simulink model "Chatr1"  (R2018b)
settings: Solver=FixedStepDiscrete  StartTime=0.0  StopTime=10.0  RelTol=1e-3
settings Model: Creator=mostafa  LastModifiedBy=mostafa
settings DataIOCC: ReturnWorkspaceOutputs=on
settings OptimizationCC: DefaultParameterBehavior=Inlined  EnhancedBackFolding=on  PassReuseOutputArgsAs=Individual arguments  ZeroExternalMemoryAtStartup=off  ZeroInternalMemoryAtStartup=off  OptimizeBlockOrder=speed  DifferentSizesBufferReuse=on  OptimizationCustomize=off
settings DebuggingCC: UnderspecifiedInitializationDetection=Classic  MergeDetectMultiDrivingBlocksExec=none  ParameterTunabilityLossMsg=error  SFMachineParentedDataDiag=error
settings ModelReferenceCC: PropagateSignalLabelsOutOfModel=off
settings SFSimCC: MATLABDynamicMemAlloc=off
settings RTWCC: SystemTargetFile=ert.tlc  GenCodeOnly=on  TemplateMakefile=ert_default_tmf  GenerateReport=on  IncludeHyperlinkInReport=on  LaunchReport=on  GenerateTraceInfo=on  GenerateTraceReport=on  GenerateTraceReportSl=on  GenerateTraceReportSf=on  GenerateTraceReportEml=on
settings CodeAppCC: ForceParamTrailComments=on  IgnoreCustomStorageClasses=off  OperatorAnnotations=on  SimulinkDataObjDesc=on  SFDataObjDesc=on  InsertBlockDesc=on  StateflowObjectComments=on
settings ERTTargetCC: TargetLangStandard=C99 (ISO)  GenerateSampleERTMain=on  InlinedParameterPlacement=NonHierarchical  ERTCustomFileTemplate=example_file_process.tlc

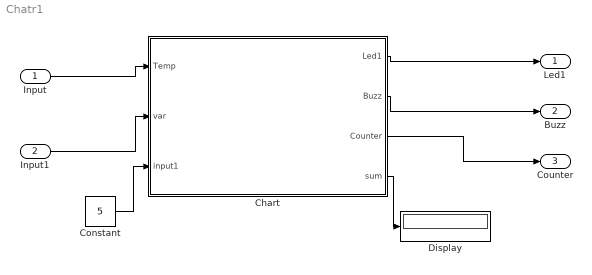
== system Chatr1 ==
  Input : Inport
  Input1 : Inport  Port=2
  Chart : Stateflow chart  TreatAsAtomicUnit=on
  Constant : Constant  Value=5  VectorParams1D=off  OutDataTypeStr=uint8
  Display : Display
  "Led1 " : Outport
  Buzz : Outport  Port=2
  Counter : Outport  Port=3
  wires:
  Chart/1(Led1) -> "Led1 "/1
  Chart/2(Buzz) -> Buzz/1
  Input/1 -> Chart/1(Temp)
  Input1/1 -> Chart/2(var)
  Chart/3(Counter) -> Counter/1
  Constant/1 -> Chart/3(input1)
  Chart/4(sum) -> Display/1

== stateflow chart Chatr1/Chart ==
  note: Do not put any code along
      | the transitions that run
      | down the right side!
  state AlarmOff [commented out]
    en:
    % initialize
    Offcounter=0;
    du:
    Led1 =0;
    Buzz=0;
    Offcounter++;
    ex:
  state AlarmOn [commented out]
    du:
    Led1=1;
    Buzz=1;
    OnCounter++;
    ex:
  (default) -> (junction 89) : /* Fact */
  (junction 90) -> (junction 88) [order 1] : [index<=input1]
  (junction 88) -> (junction 91) : {sum=sum*index;}
  (junction 89) -> (junction 90) : {index=1;sum=1;}
  (default) -> (junction 52) [commented out] : /* kareem*/
  (junction 91) -> (junction 90) : {index=index+1;}
  (junction 90) -> (junction 92) [order 2]
  (junction 52) -> (junction 53) [commented out] : [var == 1]
  (junction 52) -> (junction 56) [commented out]
  (junction 53) -> (junction 54) [commented out] : {Counter++;}
  (junction 54) -> (junction 55) [commented out]
  (junction 55) -> (junction 59) [commented out]
  (junction 56) -> (junction 57) [commented out] : [var == 2]
  (junction 56) -> (junction 60) [commented out]
  (junction 57) -> (junction 58) [commented out] : {Counter+=2;}
  (junction 58) -> (junction 59) [commented out]
  (junction 59) -> (junction 63) [commented out]
  (junction 60) -> (junction 61) [commented out] : [var == 3]
  (junction 60) -> (junction 64) [commented out] : {Counter=0;}
  (junction 61) -> (junction 62) [commented out] : {Counter+=10;}
  (junction 62) -> (junction 63) [commented out]
  (junction 63) -> (junction 65) [commented out]
  (junction 65) -> (junction 64) [commented out]
  (junction 64) -> (junction 66) [commented out]
  (default) -> AlarmOff [commented out]
  (default) -> (junction 23) [commented out] : /* Example Condition */
  AlarmOff -> AlarmOn [commented out] : [Temp>25]
  (junction 23) -> (junction 24) [commented out] : [var>100]
  (junction 23) -> (junction 25) [commented out]
  (junction 24) -> (junction 29) [commented out] : {Counter++;}
  AlarmOn -> AlarmOff [commented out] : [Temp<=25]
  (junction 25) -> (junction 26) [commented out] : [var<200]
  (junction 25) -> (junction 27) [commented out] : {Counter=0;}
  (junction 26) -> (junction 28) [commented out] : {Counter--;}
  (junction 28) -> (junction 27) [commented out]
  (junction 29) -> (junction 28) [commented out]
  (junction 27) -> (junction 30) [commented out]
  data: Led1 output uint8 [0..1] =0; Buzz output uint8; Temp input uint8; Offcounter local uint8; OnCounter local uint8; var input uint8; Counter output uint8 =0; index local uint8 =1; input1 input uint8 =5; sum output uint8 =uint8(1)
